simulink model "modelagem_2021a_2"  (R2021a)
settings: Solver=VariableStepAuto  StartTime=0.0  StopTime=10000  FixedStep=10^-6  MaxStep=10^-2  RelTol=1e-3
StopFcn:
  | q = out.logsout{2}.Values;
  | wc = out.logsout{1}.Values;
  | eul = out.logsout{3}.Values
  | figure(1)
  | plot(q.Time,q.Data)
  | legend("q0","q1","q2","q3")
  | ylabel("Quaternions")
  | xlabel("Tempo [s]")
  | hold off
  | 
  | figure(2)
  | plot(wc.Time,wc.Data)
  | legend("\omega_x","\omega_y","\omega_z")
  | ylabel("Velocidade Angular [rad/s]")
  | xlabel("Tempo [s]")
  | 
  | figure(3)
  | plot(eul.Time,eul.Data)
  | legend("\psi","\theta","\phi")
  | ylabel("Ângulos de Euler (ZYZ) [°]")
  | xlabel("Tempo [s]")
values from neighbouring files (symbols this model uses):
  b = 17.03*10^(-6)    (= 1.703e-05)    [modelagem_script.m]
  g = [0;0;-9.81]    [modelagem_script.m]
  Ic = [0.00919625 -0.00309375 -0.00225 ... (first row only)    [modelagem_script.m]
  Ic_inv = inv(Ic)    [modelagem_script.m]
  mc = 0.55    [modelagem_script.m]
  q00 = [1;0;0;0]    [modelagem_script.m]
  rc = [0.0954545;0.0954545;0.095454]    [modelagem_script.m]
  Tau = [0; 0; 0]    [modelagem_script.m]
  w00 = [0;0;0]    [modelagem_script.m]
libraries: vrlib x2
settings Model: Creator=guimi  LastModifiedBy=guimi
settings DataIOCC: SaveFinalState=on  InspectSignalLogs=on
settings DebuggingCC: UnconnectedInputMsg=none  UnconnectedOutputMsg=none  UnconnectedLineMsg=none
settings ModelReferenceCC: EnableRefExpFcnMdlSchedulingChecks=off
settings RTWCC: Description=Generic Real-Time Target  DLArmComputeVersion=20.02.1

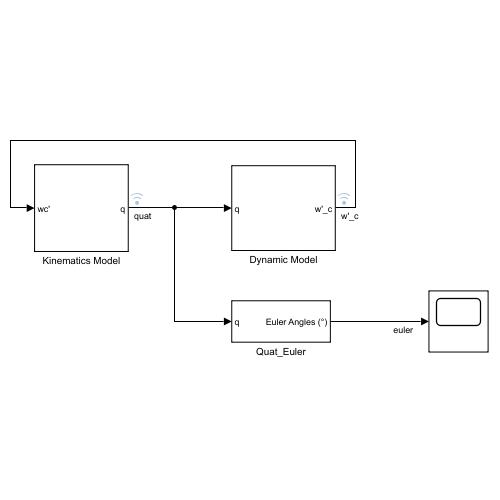
[thumbnail: Simulink's stored preview of the top-level diagram]
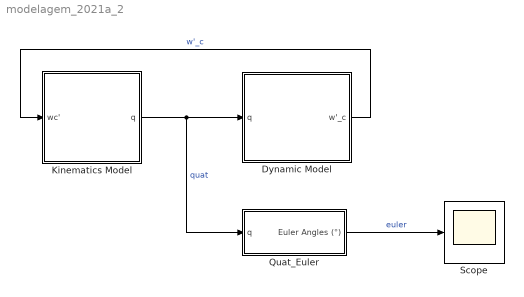
== system modelagem_2021a_2 ==
  Dynamic Model : Subsystem
  Kinematics Model : Subsystem
  Quat_Euler : Subsystem
  Scope : Scope
  wires:
  Kinematics Model/1(q) -> Quat_Euler/1(q), Dynamic Model/1(q)  "quat"
  Dynamic Model/1(w'_c) -> Kinematics Model/1(wc')  "w'_c"
  Quat_Euler/1(Euler Angles (°)) -> Scope/1  "euler"

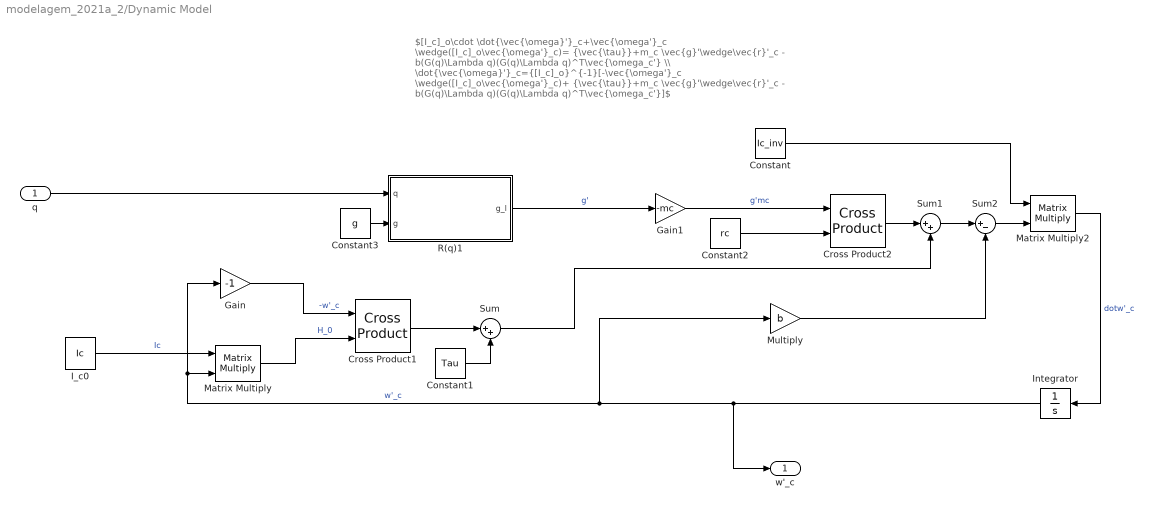
== system modelagem_2021a_2/Dynamic Model ==
  note: $[I_c]_o\cdot \dot{\vec{\omega}'}_c+\vec{\omega'}_c \wedge([I_c]_o\vec{\omega'}_c)= {\vec{\tau}}+m_c \vec{g}'\wedge\vec{r}'_c - b(G(q)\Lambda q)(G(q)\Lambda q)^T\vec{\omega_c'} \\ \dot{\vec{\omega}'}_c={[I_c]_o}^{-1}[-\vec{\omega'}_c \wedge([I_c]_o\vec{\omega'}_c)+ {\vec{\tau}}+m_c \vec{g}'\wedge\vec{r}'_c - b(G(q)\Lambda q)(G(q)\Lambda q)^T\vec{\omega_c'}]$
  q : Inport
  Constant : Constant  Value=Ic_inv
  Constant1 : Constant  Value=Tau
  Constant2 : Constant  Value=rc
  Constant3 : Constant  Value=g
  Cross Product1 : vrlib/Utilities/Cross Product
  Cross Product2 : vrlib/Utilities/Cross Product
  Gain : Gain  Gain=-1
  Gain1 : Gain  Gain=-mc
  I_c0 : Constant  Value=Ic
  Integrator : Integrator  InitialCondition=w00
  Matrix Multiply : Product  Multiplication=Matrix(*)
  Matrix Multiply2 : Product  Multiplication=Matrix(*)
  Multiply : Gain  Gain=b
  R(q)1 : MATLAB Function  TreatAsAtomicUnit=on
  Sum : Sum  Inputs=|++
  Sum1 : Sum  Inputs=|++
  Sum2 : Sum  Inputs=|+-
  w'_c : Outport
  wires:
  I_c0/1 -> Matrix Multiply/1  "Ic"
  Integrator/1 -> Matrix Multiply/2, Gain/1, Multiply/1, w'_c/1  "w'_c"
  Matrix Multiply/1 -> Cross Product1/2  "H_0"
  Gain/1 -> Cross Product1/1  "-w'_c"
  Cross Product1/1 -> Sum/1
  Constant1/1 -> Sum/2
  q/1 -> R(q)1/1(q)
  Gain1/1 -> Cross Product2/1  "g'mc"
  Constant2/1 -> Cross Product2/2
  Sum/1 -> Sum1/2
  Sum1/1 -> Sum2/1
  Multiply/1 -> Sum2/2
  Sum2/1 -> Matrix Multiply2/2
  Constant/1 -> Matrix Multiply2/1
  Matrix Multiply2/1 -> Integrator/1  "dotw'_c"
  Cross Product2/1 -> Sum1/1
  R(q)1/1(g_l) -> Gain1/1  "g'"
  Constant3/1 -> R(q)1/2(g)

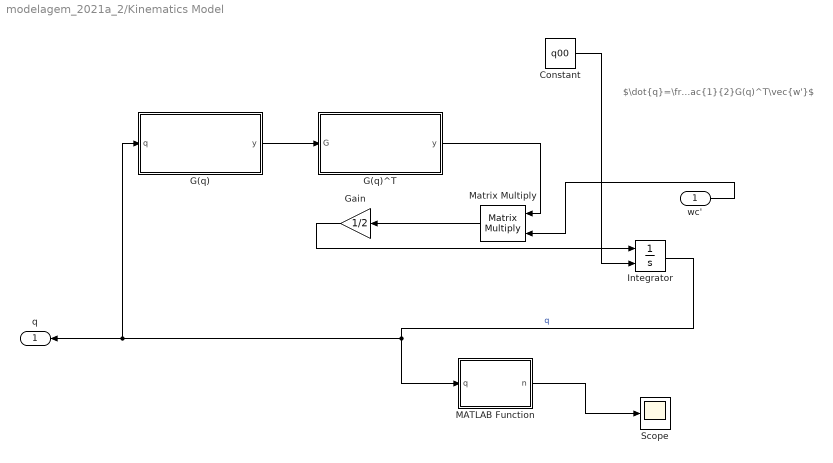
== system modelagem_2021a_2/Kinematics Model ==
  note: $\dot{q}=\frac{1}{2}G(q)^T\vec{w'}$
  wc' : Inport
  Constant : Constant  Value=q00
  G(q) : MATLAB Function  TreatAsAtomicUnit=on
  G(q)^T : MATLAB Function  TreatAsAtomicUnit=on
  Gain : Gain  Gain=1/2
  Integrator : Integrator  InitialConditionSource=external  InitialCondition=q00  UpperSaturationLimit=1  LowerSaturationLimit=-1
  MATLAB Function : MATLAB Function  TreatAsAtomicUnit=on
  Matrix Multiply : Product  Multiplication=Matrix(*)
  Scope : Scope
  q : Outport
  wires:
  G(q)/1(y) -> G(q)^T/1(G)
  wc'/1 -> Matrix Multiply/2
  G(q)^T/1(y) -> Matrix Multiply/1
  Integrator/1 -> MATLAB Function/1(q), G(q)/1(q), q/1  "q"
  Matrix Multiply/1 -> Gain/1
  Constant/1 -> Integrator/2
  Gain/1 -> Integrator/1
  MATLAB Function/1(n) -> Scope/1

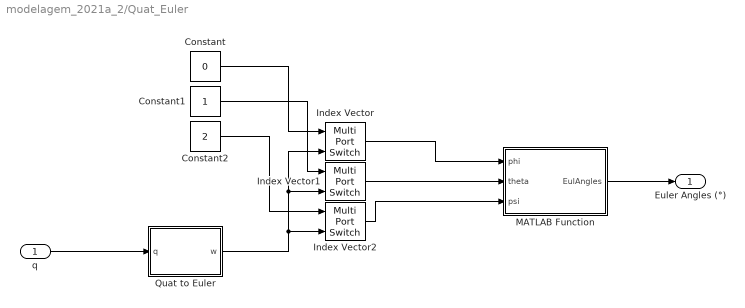
== system modelagem_2021a_2/Quat_Euler ==
  q : Inport
  Constant : Constant  Value=0
  Constant1 : Constant
  Constant2 : Constant  Value=2
  Index Vector : MultiPortSwitch  DataPortOrder=Zero-based contiguous  Inputs=1  zeroidx=on
  Index Vector1 : MultiPortSwitch  DataPortOrder=Zero-based contiguous  Inputs=1  zeroidx=on
  Index Vector2 : MultiPortSwitch  DataPortOrder=Zero-based contiguous  Inputs=1  zeroidx=on
  MATLAB Function : MATLAB Function  TreatAsAtomicUnit=on
  Quat to Euler : MATLAB Function  TreatAsAtomicUnit=on
  Euler Angles (°) : Outport
  wires:
  q/1 -> Quat to Euler/1(q)
  Quat to Euler/1(w) -> Index Vector/2, Index Vector1/2, Index Vector2/2
  Constant2/1 -> Index Vector2/1
  Constant1/1 -> Index Vector1/1
  Constant/1 -> Index Vector/1
  MATLAB Function/1(EulAngles) -> Euler Angles (°)/1
  Index Vector1/1 -> MATLAB Function/2(theta)
  Index Vector2/1 -> MATLAB Function/3(psi)
  Index Vector/1 -> MATLAB Function/1(phi)

== matlab function modelagem_2021a_2/Dynamic Model/R(q)1 ==
  data: q input; g_l output; g input
function g_l = fcn(q,g)
    I = eye(3);
    qi = [q(2);q(3);q(4)];
    qT = qi.';
    g_l = 2*dot(qi,g)*qi + q(1)^2*g + 2*q(1)*cross(g,qi) - dot(qi,qi)*g;
end

== matlab function modelagem_2021a_2/Quat_Euler/MATLAB Function ==
  data: phi input; EulAngles output; theta input; psi input
function EulAngles  = fcn(phi, theta, psi)

dphi = 180/pi *phi;
dtheta = 180/pi *theta;
dpsi = 180/pi *psi;
EulAngles = [dphi;dtheta;dpsi];
end

== matlab function modelagem_2021a_2/Quat_Euler/Quat to Euler ==
  data: q input; w output
function w = fcn(q)

    phi = atan2(q(4),q(1)) - atan2(-q(2),q(3));
    theta = acos((2*(q(1)^2+q(4)^2))-1);
    psi = atan2(q(4),q(1)) + atan2(-q(2),q(3));

w = [phi;theta;psi];

== matlab function modelagem_2021a_2/Kinematics Model/MATLAB Function ==
  data: q input; n output
function n = norm(q)
    n = sqrt(q(1)^2+q(2)^2+q(3)^2+q(4)^2);

== matlab function modelagem_2021a_2/Kinematics Model/G(q) ==
  data: q input; y output
function y = fcn(q)
    y = [-q(2) q(1) q(4) -q(3); -q(3) -q(4) q(1) q(2); -q(4) q(3) -q(2) q(1)];  
end

== matlab function modelagem_2021a_2/Kinematics Model/G(q)^T ==
  data: G input; y output
function y = fcn(G)
    y = G.';  
end
